simulink model "APA_Ncancel"  (R2024b)
settings: Solver=VariableStepAuto  StartTime=0.0  StopTime=inf  RelTol=1e-3
libraries: dspsnks4 x2, commchan3 x1, dspvision x1, dspadpt3 x1, dspsrcs4 x1
settings Model: Creator=tamiz  LastModifiedBy=tamiz

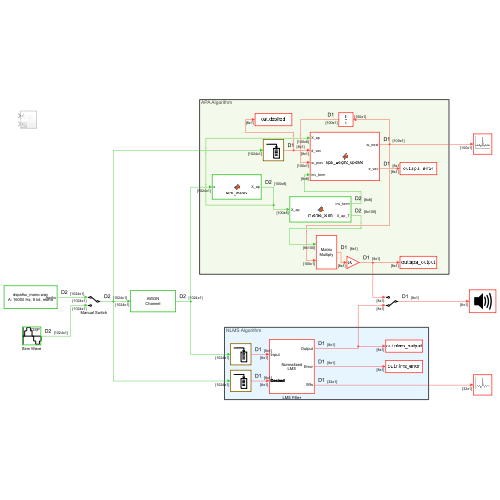
[thumbnail: Simulink's stored preview of the top-level diagram]
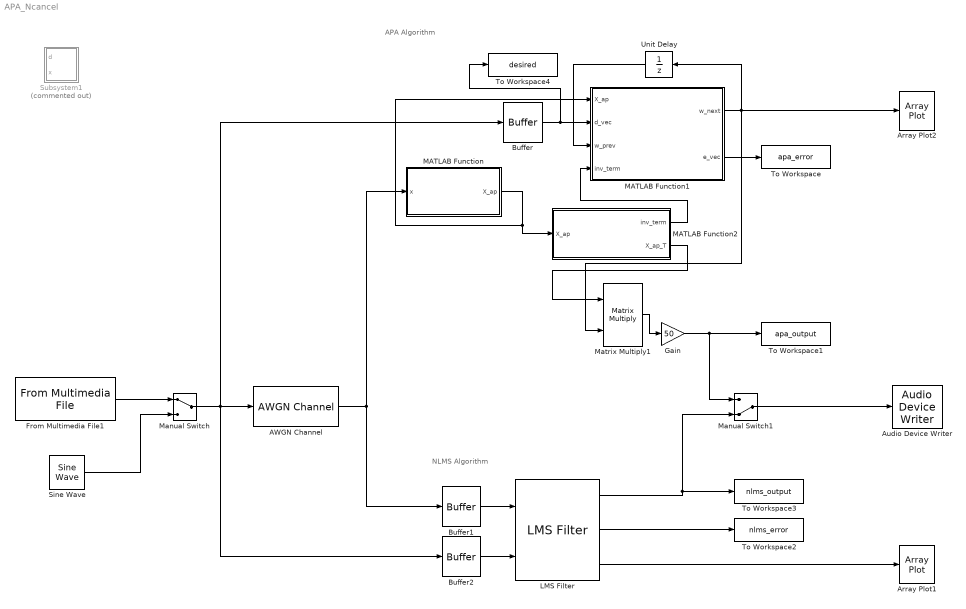
== system APA_Ncancel ==
  note: NLMS Algorithm
  note: APA Algorithm
  AWGN Channel : commchan3/AWGN Channel  LegacyMode=off  NoiseMethod="Signal to noise ratio  (SNR)"  noiseMode="Signal to noise ratio  (SNR)"  EbNo=10  EsNo=10  SNR=50  BitsPerSymbol=1  SignalPower=1  SamplesPerSymbol=1  SymbolPeriod=1  VarianceSource=Parameter  Variance=1  RandomStream=Global stream  Seed=67  SimulateUsing=Code generation
  Array Plot1 : ArrayPlot  WindowPosition=[311.000000,280.000000,800.000000,500.000000,]  ScopeFrameLocation=window  YLimits=[-0.0346 0.1518]
      settings: OpenAtSimulationStart=off
  Array Plot2 : ArrayPlot  WindowPosition=[311.000000,280.000000,800.000000,500.000000,]  ScopeFrameLocation=window  YLimits=[-0.0044 0.0061]
      settings: OpenAtSimulationStart=off
  Audio Device Writer : dspsnks4/Audio Device Writer  Driver=DirectSound  Device=Default  InheritSampleRate=on  SampleRate=44100  BitDepth=16-bit integer  BufferSize=4096  NumBuffers=10  DefaultOutputChannelMapping=on  OutputChannelMapping=1:2  OutputNumUnderrunSamples=off  DriverIdx=1  DeviceWarnFlag=''
  Buffer : Buffer  N=8  V=7  OutputFrames=off
  Buffer1 : Buffer  N=8  V=7  OutputFrames=off
  Buffer2 : Buffer  N=8  V=7  OutputFrames=off
  From Multimedia File1 : dspvision/From Multimedia File  inputFilename=C:\Program Files\MATLAB\R2024b\toolbox\dsp\dsp\samples\dspafsx_mono.wav  readRange=[1 Inf]  loop=on  numPlays=inf  outputStreams=Audio only  videoDataType=single  audioDataType=double  inheritSampleTime=on  userDefinedSampleTime=1/30  noAudioOutput=off  isIntensityVideo=off  fourcc=RGB  colorVideoFormat=Separate color signals  outputEOF=off  dataOrg=Column-major  audioFrameSize=1024  computeAudioFrameSize=off  outSamplingMode=Sample based
      settings: LibrarySourceBlock=audiosources/From Multimedia File
  Gain : Gain  Gain=50
  LMS Filter : dspadpt3/LMS Filter  Algo=Normalized LMS  L=32  stepflag=Dialog  mu=0.01  leakage=1.0  ic=0  Adapt=off  resetflag=None  weights=on  addnparflag=off  roundingMode=Floor  overflowMode=off  secondCoeffMode=Binary point scaling  secondCoeffWordLength=2  secondCoeffFracLength=15  prodOutput2Mode=Binary point scaling  prodOutput2FracLength=20  prodOutput3Mode=Binary point scaling  prodOutput3FracLength=20  prodOutput4Mode=Binary point scaling  prodOutput4FracLength=20  quotientMode=Binary point scaling  quotientFracLength=20  accum2Mode=Binary point scaling  accum2FracLength=20
      settings: LibrarySourceBlock=dsphdlsupportfiltering/LMS Filter
  MATLAB Function : MATLAB Function  TreatAsAtomicUnit=on
  MATLAB Function1 : MATLAB Function  TreatAsAtomicUnit=on
  MATLAB Function2 : MATLAB Function  TreatAsAtomicUnit=on
  Manual Switch : ManualSwitch
  Manual Switch1 : ManualSwitch  CurrentSetting=0
  Matrix Multiply1 : Product  Multiplication=Matrix(*)
  Sine Wave : dspsrcs4/Sine Wave  Amplitude=1  Frequency=1000  Phase=0  SampleMode=Discrete  OutComplex=Real  CompMethod=Trigonometric fcn  TableSize=Speed  SampleTime=1/16000  SamplesPerFrame=1024  ResetState=Restart at time zero  OutputFrames=off  dataType=double  wordLen=16  udDataType=sfix(16)  fracBitsMode=Best precision  numFracBits=15  OutDataTypeStr=double  LastOutDataTypeStr=double
  Subsystem1 : Subsystem  Commented=on
  To Workspace : ToWorkspace  VariableName=apa_error  SampleTime=-1
      settings: Save2DSignal=2-D array (concatenate along first dimension)
  To Workspace1 : ToWorkspace  VariableName=apa_output  SampleTime=-1
      settings: Save2DSignal=2-D array (concatenate along first dimension)
  To Workspace2 : ToWorkspace  VariableName=nlms_error  SampleTime=-1
      settings: Save2DSignal=2-D array (concatenate along first dimension)
  To Workspace3 : ToWorkspace  VariableName=nlms_output  SampleTime=-1
      settings: Save2DSignal=2-D array (concatenate along first dimension)
  To Workspace4 : ToWorkspace  VariableName=desired  SampleTime=-1
      settings: Save2DSignal=2-D array (concatenate along first dimension)
  Unit Delay : UnitDelay  SampleTime=-1  HasFrameUpgradeWarning=on
  wires:
  Sine Wave/1 -> Manual Switch/2
  From Multimedia File1/1 -> Manual Switch/1
  Manual Switch1/1 -> Audio Device Writer/1
  MATLAB Function1/1(w_next) -> Array Plot2/1, Matrix Multiply1/2, Unit Delay/1
  Buffer/1 -> To Workspace4/1, MATLAB Function1/2(d_vec)
  Unit Delay/1 -> MATLAB Function1/3(w_prev)
  MATLAB Function2/2(X_ap_T) -> Matrix Multiply1/1
  MATLAB Function1/2(e_vec) -> To Workspace/1
  MATLAB Function/1(X_ap) -> MATLAB Function1/1(X_ap), MATLAB Function2/1(X_ap)
  MATLAB Function2/1(inv_term) -> MATLAB Function1/4(inv_term)
  LMS Filter/1 -> To Workspace3/1, Manual Switch1/2
  LMS Filter/3 -> Array Plot1/1
  Buffer1/1 -> LMS Filter/1
  LMS Filter/2 -> To Workspace2/1
  Buffer2/1 -> LMS Filter/2
  AWGN Channel/1 -> Buffer1/1, MATLAB Function/1(x)
  Manual Switch/1 -> Buffer2/1, Buffer/1, AWGN Channel/1
  Matrix Multiply1/1 -> Gain/1
  Gain/1 -> To Workspace1/1, Manual Switch1/1

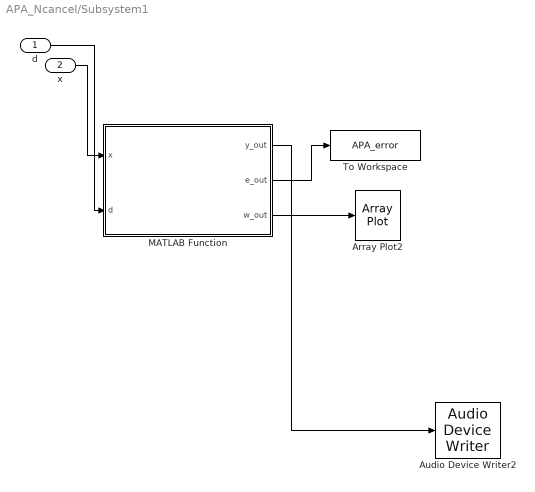
== system APA_Ncancel/Subsystem1 ==
  d : Inport
  x : Inport  Port=2
  Array Plot2 : ArrayPlot  WindowPosition=[311.000000,280.000000,800.000000,500.000000,]  ScopeFrameLocation=window  YLimits=[-0.3037538335866732 0.42849437547570246]
      settings: OpenAtSimulationStart=off
  Audio Device Writer2 : dspsnks4/Audio Device Writer  Driver=DirectSound  Device=Default  InheritSampleRate=on  SampleRate=44100  BitDepth=16-bit integer  BufferSize=4096  NumBuffers=10  DefaultOutputChannelMapping=on  OutputChannelMapping=1:2  OutputNumUnderrunSamples=off  DriverIdx=1  DeviceWarnFlag=''
  MATLAB Function : MATLAB Function  TreatAsAtomicUnit=on
  To Workspace : ToWorkspace  VariableName=APA_error  SampleTime=-1
      settings: Save2DSignal=2-D array (concatenate along first dimension)
  wires:
  MATLAB Function/1(y_out) -> Audio Device Writer2/1
  MATLAB Function/2(e_out) -> To Workspace/1
  d/1 -> MATLAB Function/2(d)
  x/1 -> MATLAB Function/1(x)
  MATLAB Function/3(w_out) -> Array Plot2/1

== matlab function APA_Ncancel/MATLAB Function1 ==
  data: X_ap input; w_next output; d_vec input; w_prev input; inv_term input; e_vec output
function [w_next, e_vec] = apa_weight_update(X_ap, d_vec, w_prev, inv_term)
% Inputs:
% X_ap     : [M x P] input data matrix
% d_vec    : [P x 1] desired signal vector
% w_prev   : [M x 1] previous weights (not used, retained for compatibility)
% inv_term : [P x P] inverse matrix: (X_ap' * X_ap + εI)^(-1)

% === Constants ===
mu = 0.01;

% === Initialize weights on first call ===
persistent w
if isempty(w)
    w = ones(size(X_ap, 1), 1);  % Initialize to [M x 1] zero vector
end

% === Compute error ===
e_vec = d_vec - X_ap' * w;  % [P x 1]

% === Weight update ===
w = w + mu * X_ap * inv_term * e_vec;  % [M x 1]

% === Outputs ===
w_next = w;

== matlab function APA_Ncancel/MATLAB Function ==
  data: x input; X_ap output
function X_ap = APA_matrix(x)
% x: input signal vector (column), size [N x 1]

% === Default Parameters ===
M = 100;      % Filter length
P = 8;
% === Current time step ===
k = length(x);  % Assume latest sample is at the end

% === Preallocate APA matrix ===
X_ap = zeros(M, P);

% === Check for valid indexing ===
if k < M + P - 1
    return; % Return zero matrix if insufficient data
end

% === Construct APA matrix ===
for i = 1:P
    idx_start = k - (i-1) - M + 1;
    idx_end = k - (i-1);
    X_ap(:, P-i+1) = x(idx_start:idx_end);
end

== matlab function APA_Ncancel/MATLAB Function2 ==
  data: X_ap input; inv_term output; X_ap_T output
function [inv_term, X_ap_T] = inverse_term(X_ap)
% Inputs:
% X_ap    : [M x P] APA input matrix
% epsilon : Regularization constant (e.g., 1e-3)

% Outputs:
% inv_term : [P x P] Inverse term (X_ap' * X_ap + εI)^(-1)
% X_ap_T   : [P x M] Transpose of X_ap

% === Compute transpose ===
X_ap_T = X_ap';
epsilon = 1e-3;
% === Compute inverse term ===
P = size(X_ap, 2);
inv_term = (X_ap_T * X_ap + epsilon * eye(P)) \ eye(P);

== matlab function APA_Ncancel/Subsystem1/MATLAB Function ==
  data: x input; y_out output; d input; e_out output; w_out output
function [y_out, e_out, w_out] = APA_main(x, d)
% Inputs:
% x     : input noisy signal [N x 1]
% d     : desired clean signal [N x 1]

% Outputs:
% y_out : APA output signal [N x 1]
% e_out : error signal [N x 1]
% w_out : final filter weights [M x 1]

% === Parameters ===
M = 32;       % Filter length
P = 8;        % Projection order
mu = 0.01;    % Step size
epsilon = 1e-3; % Regularization

% === Initialization ===
N = length(x);
w = zeros(M, 1);              % Initial weight vector
y_out = zeros(N, 1);          % Output signal
e_out = zeros(N, 1);          % Error signal

% === Processing Loop ===
for k = M+P-1:N
    % --- Construct APA input matrix X_ap [M x P] ---
    X_ap = zeros(M, P);
    for i = 1:P
        idx = k - (i-1) - M + 1 : k - (i-1);
        X_ap(:, P-i+1) = x(idx);
    end

    % --- Construct desired signal vector d_vec [P x 1] ---
    d_vec = d(k:-1:k-P+1);

    % --- Inverse term ---
    X_ap_T = X_ap';
    inv_term = (X_ap_T * X_ap + epsilon * eye(P)) \ eye(P);

    % --- APA Output and Error ---
    y_vec = X_ap_T * w;       % [P x 1]
    e_vec = d_vec - y_vec;    % [P x 1]

    % --- Update Weights ---
    w = w + mu * X_ap * inv_term * e_vec;

    % --- Save output (only use most recent estimate) ---
    y_out(k) = y_vec(1);
    e_out(k) = e_vec(1);
end

% Final weights
w_out = w;
